simulink model "Fig532"  (R2014b)
settings: Solver=ode3  StartTime=0.0  StopTime=0.1  FixedStep=1e-7  RelTol=1e-5
libraries: commofdm x1, commrandsrc2 x1
settings Model: Creator=Dennis Silage  LastModifiedBy=Silage
settings DataIOCC: SignalLoggingSaveFormat=ModelDataLogs
settings OptimizationCC: ExpressionDepthLimit=2147483647  InitFltsAndDblsToZero=on
settings DebuggingCC: UnderspecifiedInitializationDetection=Classic  MergeDetectMultiDrivingBlocksExec=none  SolverPrmCheckMsg=none  MultiTaskCondExecSysMsg=warning  MultiTaskRateTransMsg=warning  FcnCallInpInsideContextMsg=UseLocalSettings  StateNameClashWarn=warning
settings GRTTargetCC: CombineOutputUpdateFcns=off  GRTInterface=on

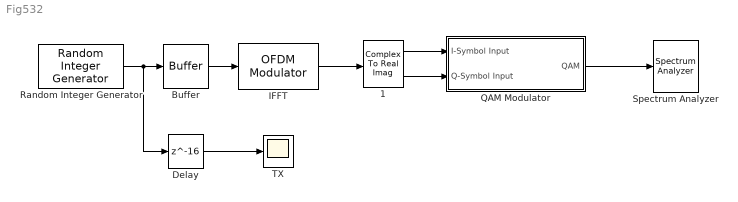
== system Fig532 ==
  "   IFFT " : commofdm/OFDM Modulator  SimulateUsing=Interpreted execution  FFTLength=8  NumGuardBandCarriers=[0 ; 0]  InsertDCNull=off  PilotInputPort=off  PilotCarrierIndices=[12; 26; 40; 54]  CyclicPrefixLength=0  Windowing=off  WindowLength=1  NumSymbols=1  NumTransmitAntennas=1
  "  1" : ComplexToRealImag  SampleTime=1e-3
  Buffer : Buffer  N=8  TreatMby1Signals=One channel
  Delay : Delay  DelayLength=16  InitialCondition=0
  QAM Modulator : Subsystem
  Random Integer Generator : commrandsrc2/Random Integer Generator  mul=2  seed=randseed  Ts=1e-3  frameBased=off  sampPerFrame=50  orient=on  outDataType=double
  Spectrum Analyzer : SpectrumAnalyzer
  TX : Scope
      settings: YMin=-8  YMax=8  SaveName=ScopeData2
  wires:
  Random Integer Generator/1 -> Delay/1, Buffer/1
  Buffer/1 -> "   IFFT "/1
  Delay/1 -> TX/1
  "  1"/1 -> QAM Modulator/1(I-Symbol Input)
  "  1"/2 -> QAM Modulator/2(Q-Symbol Input)
  "   IFFT "/1 -> "  1"/1
  QAM Modulator/1(QAM) -> Spectrum Analyzer/1

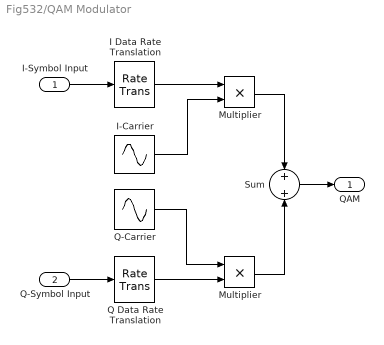
== system Fig532/QAM Modulator ==
  I-Symbol Input : Inport
  Q-Symbol Input : Inport  Port=2
  " Multiplier " : Product  RndMeth=Zero
  I Data Rate Translation : RateTransition  OutPortSampleTime=2e-6
  I-Carrier : Sin  Amplitude=5  Frequency=40000*pi  Phase=pi/2  SampleTime=2e-6  VectorParams1D=off
  Multiplier : Product  RndMeth=Zero
  Q Data Rate Translation : RateTransition  OutPortSampleTime=2e-6
  Q-Carrier : Sin  Amplitude=5  Frequency=40000*pi  SampleTime=2e-6  VectorParams1D=off
  Sum : Sum
  QAM : Outport
  wires:
  I Data Rate Translation/1 -> Multiplier/1
  Q Data Rate Translation/1 -> " Multiplier "/2
  I-Carrier/1 -> Multiplier/2
  Q-Carrier/1 -> " Multiplier "/1
  Multiplier/1 -> Sum/1
  " Multiplier "/1 -> Sum/2
  Sum/1 -> QAM/1
  I-Symbol Input/1 -> I Data Rate Translation/1
  Q-Symbol Input/1 -> Q Data Rate Translation/1
